simulink model "VehicleDynamics3D_old"  (R2018a)
settings: Solver=ode15s  StartTime=0.0  StopTime=Stoptime  FixedStep=.001  MaxStep=maxStep  RelTol=relTol  AbsTol=absTol  EnableMultiTasking=on
PreLoadFcn:
  | VehicleDynamicsInitialization.m
model workspace: external: MATLAB File C:\Users\Puspita\Desktop\VehicleDynamics\sm_suspension_templates_params_ori.m (data not in the file)
values from neighbouring files (symbols this model uses):
  contactDamping = 1200    [VehicleDynamicsInitialization.m]    (also in traj1_results.mat)
  contactStiffness = 1E+6    (= 1000000)    [VehicleDynamicsInitialization.m]    (also in traj1_results.mat)
  dwb =     [modelworkspace.mat]    (also in sm_suspension_templates_params_ref.m = struct)
  Floor =     [traj1_results.mat]
  followerCameraX = 7.5    [VehicleDynamicsInitialization.m]    (also in traj1_results.mat)
  followerCameraZ = 3    [VehicleDynamicsInitialization.m]    (also in traj1_results.mat)
  frontCameraX = -1.75    [VehicleDynamicsInitialization.m]    (also in traj1_results.mat)
  frontCameraZ = 0.35    [VehicleDynamicsInitialization.m]    (also in traj1_results.mat)
  isoCameraAimX = (1/2)*wheelbase    (= 0.75)    [VehicleDynamicsInitialization.m]    (also in traj1_results.mat)
  isoCameraX = -3.1    [VehicleDynamicsInitialization.m]    (also in traj1_results.mat)
  isoCameraY = 3.5    [VehicleDynamicsInitialization.m]    (also in traj1_results.mat)
  isoCameraZ = 1.5    [VehicleDynamicsInitialization.m]    (also in traj1_results.mat)
  kineticFrictionCoeff = 0.88    [VehicleDynamicsInitialization.m]    (also in traj1_results.mat)
  limit = 105    [Run_Rear_Ident.m]    (also in test_traj.m = 50; traj1_results.mat = 50)
  Load = 200*scale    (= 200)    [VehicleDynamicsInitialization.m]    (also in traj1_results.mat)
  m = 200    [test_2.mat]    (also in test_traj.mat; test_traj2.mat; traj1_results.mat; traj_8.mat)
  maxSteeringDisplacement = 12    [VehicleDynamicsInitialization.m]    (also in traj1_results.mat = 10)
  minSteeringDisplacement = -12    [VehicleDynamicsInitialization.m]    (also in traj1_results.mat = -10)
  SetPaceSampleTime = 0.1    [VehicleDynamicsInitialization.m]    (also in traj1_results.mat)
  staticFrictionCoeff = 0.90    (= 0.9)    [VehicleDynamicsInitialization.m]    (also in traj1_results.mat)
  steer_input_max = 10    [Run.m]    (also in Run_Front_Ident.m; Run_Rear_Ident.m = save_array(i,1); Run_Rear_Ident2.m)
  steering_step = 7.5/30    (= 0.25)    [Run.m]    (also in Run_Front_Ident.m; Run_Rear_Ident.m; Run_Rear_Ident2.m)
  steeringInput = 0    [VehicleDynamicsInitialization.m]    (also in traj1_results.mat)
  vehicleSpeed_kph = 0    [VehicleDynamicsInitialization.m]    (also in traj1_results.mat)
  velocityThreshold = 1.5    [VehicleDynamicsInitialization.m]    (also in traj1_results.mat)
  vx_input = vx_choice(i)    [Run.m]    (also in Run_Front_Ident.m; Run_Rear_Ident.m = save_array(i,2); Run_Rear_Ident2.m)
  wheel =     [modelworkspace.mat]    (also in sm_suspension_templates_params_ref.m = struct; traj1_results.mat)
  wheelbase = 1.5*scale    (= 1.5)    [VehicleDynamicsInitialization.m]    (also in traj1_results.mat)
undefined symbols (not defined in the file or in its folder): sigbuilder_block, X, Y, Z
libraries: sm_lib x235, nesl_utility x78, sm_suspension_templates_lib x34, Contact_Forces_Lib x16, simulink x12, fl_lib x1, aerolibanimutils x1
(part 7 of 10)

== system VehicleDynamics3D_old/WheelFR/FrontRightWeelContact ==
  Bus Selector : BusSelector  OutputSignals=Normal Force,Friction Force
  Demux : Demux  Outputs=2
  Math Function : Math  Operator=square  SaturateOnIntegerOverflow=on
  Rigid Transform : sm_lib/Frames and Transforms/Rigid Transform  TranslationMethod=StandardAxis  TranslationStandardOffset=-wheel.tire.outerradius*.01  TranslationLengthUnit=m  TranslationStandardAxis=+Z  TranslationCartesianOffset=[0 0 0]  TranslationROffset=0  TranslationROffsetUnits=m  TranslationZOffset=0  TranslationZOffsetUnits=m  TranslationThetaOffset=0  TranslationThetaOffsetUnits=deg  RotationMethod=None  RotationAngleUnits=deg  RotationStandardAxis=+Z  RotationAngle=0  RotationArbitraryAxis=[0 0 1]  FollAlignAxisA=+X  BaseAlignAxisA=-X  FollAlignAxisB=+Z  BaseAlignAxisB=+Z  RotationSequenceAxes=FollowerAxes  RotationSequence=XYX  RotationSequenceAngles=[0 0 0]  RotationSequenceAnglesUnits=deg  RotationMatrix=[1 0 0; 0 1 0; 0 0 1]
  Signal Conversion : SignalConversion  OverrideOpt=off
  Signal Conversion1 : SignalConversion  OverrideOpt=off
  Sphere to Plane Force : Subsystem  AncestorBlock=Contact_Forces_Lib/3D/Sphere to Plane Force  mask(Sphere to Plane Force){sphere_rad=wheel.tire.outerradius*.01, plane_lenx=Floor.l, plane_leny=Floor.w, plane_depth=Floor.h/2, force_law=Linear, k_contact=contactStiffness, b_contact=contactDamping, pen_full_damp_F=1e-4, pen_exponent=1, custom_param_1=1, custom_param_2=1, friction_law=Stick-Slip Continuous, mu_kinetic=kineticFrictionCoeff, mu_static=staticFrictionCoeff, v_thr=velocityThreshold, vis_on=off, vis_opc_en=0, vis_len_plaBz=0.005, vis_clr=[0.9 0.2 0.2], vis_opc=0.7}
      mask prompts: sphere_rad "Sphere Radius (m)"; plane_lenx "Plane Length x (m)"; plane_leny "Plane Length y (m)"; plane_depth "Plane Depth to Reference Frame (m)"; force_law "Force Law"; k_contact "Contact Stiffness (N/m)"; b_contact "Contact Damping (N/(m/s))"; pen_full_damp_F "Penetration for full damping (m)"; pen_exponent "Penetration exponent (>=1)"; custom_param_1 "Custom Parameter 1"; custom_param_2 "Custom Parameter 2"; friction_law "Friction Law"; mu_kinetic "Coefficient of Kinetic Friction"; mu_static "Coefficient of Static Friction"; v_thr "Velocity Threshold (m/s)"; vis_on "Visualize Contact Surfaces"; vis_opc_en "Visualize Opacity Enable"; vis_len_plaBz "Depth Plane Surface Element (Z-Axis) (m)"; vis_clr "Color of Surface Element (RGB)"; vis_opc "Opacity of Surface Element (0-1)"
      mask help:
      | This subsystem implements a contact force between a sphere and a plane.  The force is active above and below the plane.
      |
      | Frame connected to PlaB port:
      | 1. Located at midpoint of plane (x, y, and z).
      | 2. Z-axis is normal to the surfaces where force is active.
      |
      | Frame connected to the SphF port:
      | 1. Located at center of sphere.
      | 2. Orientation does not matter.
      |
      | Output signal is a bus with intermediate calculations and total force. Click Help for a diagram describing this force.
      mask init: same as VehicleDynamics3D_old/WheelFL/FrontLeftWeelContact/Sphere to Plane Force
      mask Help: web(which('Sphere_to_Plane_Contact.html'));
      mask TypeOptions force_law: Linear | Nonlinear | Custom
      mask Callback force_law:
      | %maskStr = get_param(gcb,'MaskValues');
      | maskObj = Simulink.Mask.get(gcb);
      | pfd_h = maskObj.getParameter('pen_full_damp_F');
      | pex_h = maskObj.getParameter('pen_exponent');
      | cc1_h = maskObj.getParameter('custom_param_1');
      | cc2_h = maskObj.getParameter('custom_param_2');
      | if strcmp(get_param(gcb,'force_law'),'Linear')
      |     pfd_h.Visible = 'off';
      |     pex_h.Visible = 'off';
      |     cc1_h.Visible = 'off';
      |     cc2_h.Visible = 'off';
      | %    set_param(gcb,'MaskVisibilities',{'on' 'on' 'on' 'on' 'on' 'off' 'off' 'off' 'off'});
      | %    set_param(gcb,'MaskVisibilities',{'on' 'on' 'on' 'on' 'on' 'off' 'off' 'off' 'off'});
      | elseif strcmp(get_param(gcb,'force_law'),'Nonlinear')
      |     pfd_h.Visible = 'on';
      |     pex_h.Visible = 'on';
      |     cc1_h.Visible = 'off';
      |     cc2_h.Visible = 'off';
      |     %set_param(gcb,'MaskVisibilities',{'on' 'on' 'on' 'on' 'on' 'on' 'on' 'off' 'off'});
      | elseif strcmp(get_param(gcb,'force_law'),'Custom')
      |     pfd_h.Visible = 'off';
      |     pex_h.Visible = 'off';
      |     cc1_h.Visible = 'on';
      |     cc2_h.Visible = 'on';
      |     %set_param(gcb,'MaskVisibilities',{'on' 'on' 'on' 'on' 'on' 'off' 'off' 'on' 'on'});
      | end
      | %clear maskObj
      | 
      | %maskObj = Simulink.Mask.get(gcb);
      | %if strcmp(get_param(gcb,'x'),'on')
      | %else
      | %    yh.Visible = 'off';
      | %end
      mask TypeOptions friction_law: None | Stick-Slip Continuous
      mask Callback friction_law:
      | maskObj = Simulink.Mask.get(gcb);
      | muk_h = maskObj.getParameter('mu_kinetic');
      | mus_h = maskObj.getParameter('mu_static');
      | vth_h = maskObj.getParameter('v_thr');
      | if strcmp(get_param(gcb,'friction_law'),'None')
      |     muk_h.Visible = 'off';
      |     mus_h.Visible = 'off';
      |     vth_h.Visible = 'off';
      | elseif strcmp(get_param(gcb,'friction_law'),'Stick-Slip Continuous')
      |     muk_h.Visible = 'on';
      |     mus_h.Visible = 'on';
      |     vth_h.Visible = 'on';
      | end
      | clear maskObj
      mask Callback vis_on:
      | maskObj = Simulink.Mask.get(gcb);
      | vis_clr_h = maskObj.getParameter('vis_clr');
      | vis_opc_h = maskObj.getParameter('vis_opc');
      | vis_len_plaBz_h = maskObj.getParameter('vis_len_plaBz');
      | if strcmp(get_param(gcb,'vis_on'),'off')
      |     vis_len_plaBz_h.Visible = 'off';
      |     vis_clr_h.Visible = 'off';
      |     vis_opc_h.Visible = 'off';
      | elseif strcmp(get_param(gcb,'vis_on'),'on')
      |     vis_len_plaBz_h.Visible = 'on';
      |     vis_clr_h.Visible = 'on';
      |     vis_opc_h.Visible = 'on';
      | end
      | clear maskObj vis_clr_h vis_opc_h
      | clear vis_len_plaBz_h
      mask DialogControl Dim_Cont Prompt: Dimensions
      mask DialogControl Con_Cont Prompt: Contact
      mask DialogControl Fri_Cont Prompt: Friction
      mask DialogControl Container9 Prompt: Visual
      mask Display: image('Sphere_to_Plane_Contact_IMAGE.jpg');
  Sqrt : Sqrt  SaturateOnIntegerOverflow=on
  Sum of Elements : Sum  Inputs=+
  Terminator : Terminator
  Terminator1 : Terminator
  Terminator2 : Terminator
  To Workspace2 : ToWorkspace  VariableName=F_Fr  SampleTime=-1
  Conn1 : PMIOPort  Side=Right
  Conn2 : PMIOPort  Port=2  Side=Left
  wires:
  Sphere to Plane Force/1(Out) -> Bus Selector/1  "FrontRight"
  Signal Conversion1/1 -> Terminator1/1  "FrontRightFriction"
  Bus Selector/1 -> Signal Conversion/1  "<Normal Force>"
  Sum of Elements/1 -> Sqrt/1
  Signal Conversion/1 -> Terminator/1  "FrontRightTireLoad"
  Math Function/1 -> Sum of Elements/1
  Bus Selector/2 -> Demux/1, Math Function/1  "<Friction Force>"
  Sqrt/1 -> Signal Conversion1/1
  Demux/1 -> To Workspace2/1
  Demux/2 -> Terminator2/1
  connections:
  Conn1/RConn1 -- Rigid Transform/RConn1
  Sphere to Plane Force/LConn1 -- Rigid Transform/LConn1
  Conn2/RConn1 -- Sphere to Plane Force/RConn1

== system VehicleDynamics3D_old/WheelRL/RearLeftWeelContact ==
  Bus Selector : BusSelector  OutputSignals=Normal Force,Friction Force
  Demux : Demux  Outputs=2
  Math Function : Math  Operator=square  SaturateOnIntegerOverflow=on
  Rigid Transform : sm_lib/Frames and Transforms/Rigid Transform  TranslationMethod=StandardAxis  TranslationStandardOffset=-wheel.tire.outerradius*.01  TranslationLengthUnit=m  TranslationStandardAxis=+Z  TranslationCartesianOffset=[0 0 0]  TranslationROffset=0  TranslationROffsetUnits=m  TranslationZOffset=0  TranslationZOffsetUnits=m  TranslationThetaOffset=0  TranslationThetaOffsetUnits=deg  RotationMethod=None  RotationAngleUnits=deg  RotationStandardAxis=+Z  RotationAngle=0  RotationArbitraryAxis=[0 0 1]  FollAlignAxisA=+X  BaseAlignAxisA=-X  FollAlignAxisB=+Z  BaseAlignAxisB=+Z  RotationSequenceAxes=FollowerAxes  RotationSequence=XYX  RotationSequenceAngles=[0 0 0]  RotationSequenceAnglesUnits=deg  RotationMatrix=[1 0 0; 0 1 0; 0 0 1]
  Signal Conversion : SignalConversion  OverrideOpt=off
  Signal Conversion1 : SignalConversion  OverrideOpt=off
  Sphere to Plane Force : Subsystem  AncestorBlock=Contact_Forces_Lib/3D/Sphere to Plane Force  mask(Sphere to Plane Force){sphere_rad=wheel.tire.outerradius*.01, plane_lenx=Floor.l, plane_leny=Floor.w, plane_depth=Floor.h/2, force_law=Linear, k_contact=contactStiffness, b_contact=contactDamping, pen_full_damp_F=1e-4, pen_exponent=1, custom_param_1=1, custom_param_2=1, friction_law=Stick-Slip Continuous, mu_kinetic=kineticFrictionCoeff, mu_static=staticFrictionCoeff, v_thr=velocityThreshold, vis_on=off, vis_opc_en=0, vis_len_plaBz=0.005, vis_clr=[0.9 0.2 0.2], vis_opc=0.7}
      mask prompts: sphere_rad "Sphere Radius (m)"; plane_lenx "Plane Length x (m)"; plane_leny "Plane Length y (m)"; plane_depth "Plane Depth to Reference Frame (m)"; force_law "Force Law"; k_contact "Contact Stiffness (N/m)"; b_contact "Contact Damping (N/(m/s))"; pen_full_damp_F "Penetration for full damping (m)"; pen_exponent "Penetration exponent (>=1)"; custom_param_1 "Custom Parameter 1"; custom_param_2 "Custom Parameter 2"; friction_law "Friction Law"; mu_kinetic "Coefficient of Kinetic Friction"; mu_static "Coefficient of Static Friction"; v_thr "Velocity Threshold (m/s)"; vis_on "Visualize Contact Surfaces"; vis_opc_en "Visualize Opacity Enable"; vis_len_plaBz "Depth Plane Surface Element (Z-Axis) (m)"; vis_clr "Color of Surface Element (RGB)"; vis_opc "Opacity of Surface Element (0-1)"
      mask help:
      | This subsystem implements a contact force between a sphere and a plane.  The force is active above and below the plane.
      |
      | Frame connected to PlaB port:
      | 1. Located at midpoint of plane (x, y, and z).
      | 2. Z-axis is normal to the surfaces where force is active.
      |
      | Frame connected to the SphF port:
      | 1. Located at center of sphere.
      | 2. Orientation does not matter.
      |
      | Output signal is a bus with intermediate calculations and total force. Click Help for a diagram describing this force.
      mask init: same as VehicleDynamics3D_old/WheelFL/FrontLeftWeelContact/Sphere to Plane Force
      mask Help: web(which('Sphere_to_Plane_Contact.html'));
      mask TypeOptions force_law: Linear | Nonlinear | Custom
      mask Callback force_law:
      | %maskStr = get_param(gcb,'MaskValues');
      | maskObj = Simulink.Mask.get(gcb);
      | pfd_h = maskObj.getParameter('pen_full_damp_F');
      | pex_h = maskObj.getParameter('pen_exponent');
      | cc1_h = maskObj.getParameter('custom_param_1');
      | cc2_h = maskObj.getParameter('custom_param_2');
      | if strcmp(get_param(gcb,'force_law'),'Linear')
      |     pfd_h.Visible = 'off';
      |     pex_h.Visible = 'off';
      |     cc1_h.Visible = 'off';
      |     cc2_h.Visible = 'off';
      | %    set_param(gcb,'MaskVisibilities',{'on' 'on' 'on' 'on' 'on' 'off' 'off' 'off' 'off'});
      | %    set_param(gcb,'MaskVisibilities',{'on' 'on' 'on' 'on' 'on' 'off' 'off' 'off' 'off'});
      | elseif strcmp(get_param(gcb,'force_law'),'Nonlinear')
      |     pfd_h.Visible = 'on';
      |     pex_h.Visible = 'on';
      |     cc1_h.Visible = 'off';
      |     cc2_h.Visible = 'off';
      |     %set_param(gcb,'MaskVisibilities',{'on' 'on' 'on' 'on' 'on' 'on' 'on' 'off' 'off'});
      | elseif strcmp(get_param(gcb,'force_law'),'Custom')
      |     pfd_h.Visible = 'off';
      |     pex_h.Visible = 'off';
      |     cc1_h.Visible = 'on';
      |     cc2_h.Visible = 'on';
      |     %set_param(gcb,'MaskVisibilities',{'on' 'on' 'on' 'on' 'on' 'off' 'off' 'on' 'on'});
      | end
      | %clear maskObj
      | 
      | %maskObj = Simulink.Mask.get(gcb);
      | %if strcmp(get_param(gcb,'x'),'on')
      | %else
      | %    yh.Visible = 'off';
      | %end
      mask TypeOptions friction_law: None | Stick-Slip Continuous
      mask Callback friction_law:
      | maskObj = Simulink.Mask.get(gcb);
      | muk_h = maskObj.getParameter('mu_kinetic');
      | mus_h = maskObj.getParameter('mu_static');
      | vth_h = maskObj.getParameter('v_thr');
      | if strcmp(get_param(gcb,'friction_law'),'None')
      |     muk_h.Visible = 'off';
      |     mus_h.Visible = 'off';
      |     vth_h.Visible = 'off';
      | elseif strcmp(get_param(gcb,'friction_law'),'Stick-Slip Continuous')
      |     muk_h.Visible = 'on';
      |     mus_h.Visible = 'on';
      |     vth_h.Visible = 'on';
      | end
      | clear maskObj
      mask Callback vis_on:
      | maskObj = Simulink.Mask.get(gcb);
      | vis_clr_h = maskObj.getParameter('vis_clr');
      | vis_opc_h = maskObj.getParameter('vis_opc');
      | vis_len_plaBz_h = maskObj.getParameter('vis_len_plaBz');
      | if strcmp(get_param(gcb,'vis_on'),'off')
      |     vis_len_plaBz_h.Visible = 'off';
      |     vis_clr_h.Visible = 'off';
      |     vis_opc_h.Visible = 'off';
      | elseif strcmp(get_param(gcb,'vis_on'),'on')
      |     vis_len_plaBz_h.Visible = 'on';
      |     vis_clr_h.Visible = 'on';
      |     vis_opc_h.Visible = 'on';
      | end
      | clear maskObj vis_clr_h vis_opc_h
      | clear vis_len_plaBz_h
      mask DialogControl Dim_Cont Prompt: Dimensions
      mask DialogControl Con_Cont Prompt: Contact
      mask DialogControl Fri_Cont Prompt: Friction
      mask DialogControl Container9 Prompt: Visual
      mask Display: image('Sphere_to_Plane_Contact_IMAGE.jpg');
  Sqrt : Sqrt  SaturateOnIntegerOverflow=on
  Sum of Elements : Sum  Inputs=+
  Terminator : Terminator
  Terminator1 : Terminator
  Terminator2 : Terminator
  To Workspace2 : ToWorkspace  VariableName=F_Rl  SampleTime=-1
  Conn1 : PMIOPort  Side=Right
  Conn2 : PMIOPort  Port=2  Side=Left
  wires:
  Sphere to Plane Force/1(Out) -> Bus Selector/1
  Signal Conversion1/1 -> Terminator2/1  "RearLeftFriction"
  Sum of Elements/1 -> Sqrt/1
  Bus Selector/1 -> Signal Conversion/1  "<Normal Force>"
  Signal Conversion/1 -> Terminator/1  "RearLeftTireLoad"
  Math Function/1 -> Sum of Elements/1
  Sqrt/1 -> Signal Conversion1/1
  Bus Selector/2 -> Demux/1, Math Function/1  "<Friction Force>"
  Demux/1 -> To Workspace2/1
  Demux/2 -> Terminator1/1
  connections:
  Conn1/RConn1 -- Rigid Transform/RConn1
  Sphere to Plane Force/LConn1 -- Rigid Transform/LConn1
  Sphere to Plane Force/RConn1 -- Conn2/RConn1

== system VehicleDynamics3D_old/WheelRR/RearRightWeelContact ==
  Bus Selector : BusSelector  OutputSignals=Normal Force,Friction Force
  Demux : Demux  Outputs=2
  Math Function : Math  Operator=square  SaturateOnIntegerOverflow=on
  Rigid Transform : sm_lib/Frames and Transforms/Rigid Transform  TranslationMethod=StandardAxis  TranslationStandardOffset=-wheel.tire.outerradius*.01  TranslationLengthUnit=m  TranslationStandardAxis=+Z  TranslationCartesianOffset=[0 0 0]  TranslationROffset=0  TranslationROffsetUnits=m  TranslationZOffset=0  TranslationZOffsetUnits=m  TranslationThetaOffset=0  TranslationThetaOffsetUnits=deg  RotationMethod=None  RotationAngleUnits=deg  RotationStandardAxis=+Z  RotationAngle=0  RotationArbitraryAxis=[0 0 1]  FollAlignAxisA=+X  BaseAlignAxisA=-X  FollAlignAxisB=+Z  BaseAlignAxisB=+Z  RotationSequenceAxes=FollowerAxes  RotationSequence=XYX  RotationSequenceAngles=[0 0 0]  RotationSequenceAnglesUnits=deg  RotationMatrix=[1 0 0; 0 1 0; 0 0 1]
  Signal Conversion : SignalConversion  OverrideOpt=off
  Signal Conversion1 : SignalConversion  OverrideOpt=off
  Sphere to Plane Force : Subsystem  AncestorBlock=Contact_Forces_Lib/3D/Sphere to Plane Force  mask(Sphere to Plane Force){sphere_rad=wheel.tire.outerradius*.01, plane_lenx=Floor.l, plane_leny=Floor.w, plane_depth=Floor.h/2, force_law=Linear, k_contact=contactStiffness, b_contact=contactDamping, pen_full_damp_F=1e-4, pen_exponent=1, custom_param_1=1, custom_param_2=1, friction_law=Stick-Slip Continuous, mu_kinetic=kineticFrictionCoeff, mu_static=staticFrictionCoeff, v_thr=velocityThreshold, vis_on=off, vis_opc_en=0, vis_len_plaBz=0.005, vis_clr=[0.9 0.2 0.2], vis_opc=0.7}
      mask prompts: sphere_rad "Sphere Radius (m)"; plane_lenx "Plane Length x (m)"; plane_leny "Plane Length y (m)"; plane_depth "Plane Depth to Reference Frame (m)"; force_law "Force Law"; k_contact "Contact Stiffness (N/m)"; b_contact "Contact Damping (N/(m/s))"; pen_full_damp_F "Penetration for full damping (m)"; pen_exponent "Penetration exponent (>=1)"; custom_param_1 "Custom Parameter 1"; custom_param_2 "Custom Parameter 2"; friction_law "Friction Law"; mu_kinetic "Coefficient of Kinetic Friction"; mu_static "Coefficient of Static Friction"; v_thr "Velocity Threshold (m/s)"; vis_on "Visualize Contact Surfaces"; vis_opc_en "Visualize Opacity Enable"; vis_len_plaBz "Depth Plane Surface Element (Z-Axis) (m)"; vis_clr "Color of Surface Element (RGB)"; vis_opc "Opacity of Surface Element (0-1)"
      mask help:
      | This subsystem implements a contact force between a sphere and a plane.  The force is active above and below the plane.
      |
      | Frame connected to PlaB port:
      | 1. Located at midpoint of plane (x, y, and z).
      | 2. Z-axis is normal to the surfaces where force is active.
      |
      | Frame connected to the SphF port:
      | 1. Located at center of sphere.
      | 2. Orientation does not matter.
      |
      | Output signal is a bus with intermediate calculations and total force. Click Help for a diagram describing this force.
      mask init: same as VehicleDynamics3D_old/WheelFL/FrontLeftWeelContact/Sphere to Plane Force
      mask Help: web(which('Sphere_to_Plane_Contact.html'));
      mask TypeOptions force_law: Linear | Nonlinear | Custom
      mask Callback force_law:
      | %maskStr = get_param(gcb,'MaskValues');
      | maskObj = Simulink.Mask.get(gcb);
      | pfd_h = maskObj.getParameter('pen_full_damp_F');
      | pex_h = maskObj.getParameter('pen_exponent');
      | cc1_h = maskObj.getParameter('custom_param_1');
      | cc2_h = maskObj.getParameter('custom_param_2');
      | if strcmp(get_param(gcb,'force_law'),'Linear')
      |     pfd_h.Visible = 'off';
      |     pex_h.Visible = 'off';
      |     cc1_h.Visible = 'off';
      |     cc2_h.Visible = 'off';
      | %    set_param(gcb,'MaskVisibilities',{'on' 'on' 'on' 'on' 'on' 'off' 'off' 'off' 'off'});
      | %    set_param(gcb,'MaskVisibilities',{'on' 'on' 'on' 'on' 'on' 'off' 'off' 'off' 'off'});
      | elseif strcmp(get_param(gcb,'force_law'),'Nonlinear')
      |     pfd_h.Visible = 'on';
      |     pex_h.Visible = 'on';
      |     cc1_h.Visible = 'off';
      |     cc2_h.Visible = 'off';
      |     %set_param(gcb,'MaskVisibilities',{'on' 'on' 'on' 'on' 'on' 'on' 'on' 'off' 'off'});
      | elseif strcmp(get_param(gcb,'force_law'),'Custom')
      |     pfd_h.Visible = 'off';
      |     pex_h.Visible = 'off';
      |     cc1_h.Visible = 'on';
      |     cc2_h.Visible = 'on';
      |     %set_param(gcb,'MaskVisibilities',{'on' 'on' 'on' 'on' 'on' 'off' 'off' 'on' 'on'});
      | end
      | %clear maskObj
      | 
      | %maskObj = Simulink.Mask.get(gcb);
      | %if strcmp(get_param(gcb,'x'),'on')
      | %else
      | %    yh.Visible = 'off';
      | %end
      mask TypeOptions friction_law: None | Stick-Slip Continuous
      mask Callback friction_law:
      | maskObj = Simulink.Mask.get(gcb);
      | muk_h = maskObj.getParameter('mu_kinetic');
      | mus_h = maskObj.getParameter('mu_static');
      | vth_h = maskObj.getParameter('v_thr');
      | if strcmp(get_param(gcb,'friction_law'),'None')
      |     muk_h.Visible = 'off';
      |     mus_h.Visible = 'off';
      |     vth_h.Visible = 'off';
      | elseif strcmp(get_param(gcb,'friction_law'),'Stick-Slip Continuous')
      |     muk_h.Visible = 'on';
      |     mus_h.Visible = 'on';
      |     vth_h.Visible = 'on';
      | end
      | clear maskObj
      mask Callback vis_on:
      | maskObj = Simulink.Mask.get(gcb);
      | vis_clr_h = maskObj.getParameter('vis_clr');
      | vis_opc_h = maskObj.getParameter('vis_opc');
      | vis_len_plaBz_h = maskObj.getParameter('vis_len_plaBz');
      | if strcmp(get_param(gcb,'vis_on'),'off')
      |     vis_len_plaBz_h.Visible = 'off';
      |     vis_clr_h.Visible = 'off';
      |     vis_opc_h.Visible = 'off';
      | elseif strcmp(get_param(gcb,'vis_on'),'on')
      |     vis_len_plaBz_h.Visible = 'on';
      |     vis_clr_h.Visible = 'on';
      |     vis_opc_h.Visible = 'on';
      | end
      | clear maskObj vis_clr_h vis_opc_h
      | clear vis_len_plaBz_h
      mask DialogControl Dim_Cont Prompt: Dimensions
      mask DialogControl Con_Cont Prompt: Contact
      mask DialogControl Fri_Cont Prompt: Friction
      mask DialogControl Container9 Prompt: Visual
      mask Display: image('Sphere_to_Plane_Contact_IMAGE.jpg');
  Sqrt : Sqrt  SaturateOnIntegerOverflow=on
  Sum of Elements : Sum  Inputs=+
  Terminator1 : Terminator
  Terminator2 : Terminator
  Terminator3 : Terminator
  To Workspace2 : ToWorkspace  VariableName=F_Rr  SampleTime=-1
  Conn1 : PMIOPort  Side=Right
  Conn2 : PMIOPort  Port=2  Side=Left
  wires:
  Sphere to Plane Force/1(Out) -> Bus Selector/1  "RearRight"
  Bus Selector/1 -> Signal Conversion1/1  "<Normal Force>"
  Bus Selector/2 -> Demux/1, Signal Conversion/1  "<Friction Force>"
  Math Function/1 -> Sum of Elements/1
  Sum of Elements/1 -> Sqrt/1
  Sqrt/1 -> Terminator2/1  "RearRightFriction"
  Signal Conversion/1 -> Math Function/1
  Signal Conversion1/1 -> Terminator1/1  "RearRightTireLoad"
  Demux/1 -> To Workspace2/1
  Demux/2 -> Terminator3/1
  connections:
  Sphere to Plane Force/LConn1 -- Rigid Transform/LConn1
  Conn1/RConn1 -- Rigid Transform/RConn1
  Conn2/RConn1 -- Sphere to Plane Force/RConn1

== system VehicleDynamics3D_old/FrontSuspension/6DOF Motion/WraptTo180 ==
  Yaw : Inport
  Bias : Bias  Bias=-180
  Bias1 : Bias  Bias=180
  Constant : Constant  Value=360
  Interval Test : simulink/Logic and Bit Operations/Interval Test  IntervalClosedRight=on  uplimit=180  IntervalClosedLeft=off  lowlimit=-180  OutDataTypeStr=boolean
  Math Function : Math  Operator=mod  SaturateOnIntegerOverflow=on
  Switch : Switch  Criteria=u2 ~= 0
  NormalizedYaw : Outport
  wires:
  Bias1/1 -> Math Function/1
  Switch/1 -> NormalizedYaw/1  "VehicleYawNormalized_Deg"
  Constant/1 -> Math Function/2
  Interval Test/1 -> Switch/2
  Math Function/1 -> Bias/1
  Bias/1 -> Switch/3
  Yaw/1 -> Switch/1, Interval Test/1, Bias1/1

== system VehicleDynamics3D_old/FrontSuspension/Chassis Assembly/Front Frame ==
  DL XForm : sm_lib/Frames and Transforms/Rigid Transform  TranslationMethod=Cartesian  TranslationStandardOffset=0  TranslationLengthUnit=cm  TranslationStandardAxis=+Z  TranslationCartesianOffset=[swc 0]  TranslationROffset=0  TranslationROffsetUnits=m  TranslationZOffset=0  TranslationZOffsetUnits=m  TranslationThetaOffset=0  TranslationThetaOffsetUnits=deg  RotationMethod=None  RotationAngleUnits=deg  RotationStandardAxis=+Z  RotationAngle=0  RotationArbitraryAxis=[0 0 1]  FollAlignAxisA=+X  BaseAlignAxisA=-X  FollAlignAxisB=+Y  BaseAlignAxisB=-Y  RotationSequenceAxes=FollowerAxes  RotationSequence=XYX  RotationSequenceAngles=[0 0 0]  RotationSequenceAnglesUnits=deg  RotationMatrix=[1 0 0; 0 1 0; 0 0 1]
  DR XForm : sm_lib/Frames and Transforms/Rigid Transform  TranslationMethod=Cartesian  TranslationStandardOffset=0  TranslationLengthUnit=cm  TranslationStandardAxis=+Z  TranslationCartesianOffset=[sec 0]  TranslationROffset=0  TranslationROffsetUnits=m  TranslationZOffset=0  TranslationZOffsetUnits=m  TranslationThetaOffset=0  TranslationThetaOffsetUnits=deg  RotationMethod=None  RotationAngleUnits=deg  RotationStandardAxis=+Z  RotationAngle=0  RotationArbitraryAxis=[0 0 1]  FollAlignAxisA=+X  BaseAlignAxisA=+Y  FollAlignAxisB=+Y  BaseAlignAxisB=+Z  RotationSequenceAxes=FollowerAxes  RotationSequence=XYX  RotationSequenceAngles=[0 0 0]  RotationSequenceAnglesUnits=deg  RotationMatrix=[1 0 0; 0 1 0; 0 0 1]
  Frame : sm_lib/Body Elements/Solid  InertiaType=CalculateFromGeometry  Mass=1  MassUnits=kg  CenterOfMass=[0 0 0]  CenterOfMassUnits=m  MomentsOfInertia=[1 1 1]  MomentsOfInertiaUnits=kg*m^2  ProductsOfInertia=[0 0 0]  ProductsOfInertiaUnits=kg*m^2  DensityBased=on  Density=rho  DensityUnits=kg/(m^3)  DoExposeReferenceFrame=on  SerializedFrames=<Frames/>  GraphicType=FromGeometry  MarkerShape=Sphere  MarkerSize=10  MarkerSizeUnits=m  GraphicVisPropType=SimpleVisualProperties  GraphicDiffuseColor=clr  GraphicSpecularColor=[0.5 0.5 0.5 1.0]  GraphicAmbientColor=[0.15 0.15 0.15 1.0]  GraphicEmissiveColor=[0.0 0.0 0.0 1.0]  GraphicShininess=75  GraphicOpacity=1.0  GeometryShape=GeneralExtrusion  RectangleSize=[1 1]  RectangleSizeUnits=m  BrickDimensions=[1 1 1]  BrickDimensionUnits=m  CylinderRadius=1  CylinderRadiusUnits=m  CylinderLength=1  CylinderLengthUnits=m  SphereRadius=1  SphereRadiusUnits=m  EllipsoidRadii=[1 1 1]  EllipsoidRadiiUnits=m  ExtrusionCrossSection=frame_xsec  ExtrusionCrossSectionUnits=cm  ExtrusionLength=T  ExtrusionLengthUnits=cm  PolygonNumSides=3  PolygonOuterRadius=1  PolygonOuterRadiusUnits=m  ExtGeomFileType=STL  ExtGeomFileUnits=m  RevolutionCrossSection=[1 1; 1 -1; 2 -1; 2 1]  RevolutionCrossSectionUnits=m  RevolutionExtent=Full  RevolutionAngle=180  RevolutionAngleUnits=deg
  UL XForm : sm_lib/Frames and Transforms/Rigid Transform  TranslationMethod=Cartesian  TranslationStandardOffset=0  TranslationLengthUnit=cm  TranslationStandardAxis=+Z  TranslationCartesianOffset=[nwc 0]  TranslationROffset=0  TranslationROffsetUnits=m  TranslationZOffset=0  TranslationZOffsetUnits=m  TranslationThetaOffset=0  TranslationThetaOffsetUnits=deg  RotationMethod=None  RotationAngleUnits=deg  RotationStandardAxis=+Z  RotationAngle=0  RotationArbitraryAxis=[0 0 1]  FollAlignAxisA=+X  BaseAlignAxisA=-X  FollAlignAxisB=+Y  BaseAlignAxisB=-Y  RotationSequenceAxes=FollowerAxes  RotationSequence=XYX  RotationSequenceAngles=[0 0 0]  RotationSequenceAnglesUnits=deg  RotationMatrix=[1 0 0; 0 1 0; 0 0 1]
  UR XForm : sm_lib/Frames and Transforms/Rigid Transform  TranslationMethod=Cartesian  TranslationStandardOffset=0  TranslationLengthUnit=cm  TranslationStandardAxis=+Z  TranslationCartesianOffset=[nec 0]  TranslationROffset=0  TranslationROffsetUnits=m  TranslationZOffset=0  TranslationZOffsetUnits=m  TranslationThetaOffset=0  TranslationThetaOffsetUnits=deg  RotationMethod=None  RotationAngleUnits=deg  RotationStandardAxis=+Z  RotationAngle=0  RotationArbitraryAxis=[0 0 1]  FollAlignAxisA=+X  BaseAlignAxisA=+Y  FollAlignAxisB=+Y  BaseAlignAxisB=+Z  RotationSequenceAxes=FollowerAxes  RotationSequence=XYX  RotationSequenceAngles=[0 0 0]  RotationSequenceAnglesUnits=deg  RotationMatrix=[1 0 0; 0 1 0; 0 0 1]
  UL : PMIOPort  Side=Left
  DL : PMIOPort  Port=2  Side=Left
  DR : PMIOPort  Port=3  Side=Left
  UR : PMIOPort  Port=4  Side=Left
  connections:
  Frame/RConn1 -- UL XForm/LConn1 -- DL XForm/LConn1 -- DR XForm/LConn1 -- UR XForm/LConn1
  UR XForm/RConn1 -- UR/RConn1
  DL XForm/RConn1 -- DL/RConn1
  UL XForm/RConn1 -- UL/RConn1
  DR XForm/RConn1 -- DR/RConn1

== system VehicleDynamics3D_old/FrontSuspension/Chassis Assembly/Load ==
  Chassis Load : sm_lib/Body Elements/Solid  InertiaType=PointMass  Mass=Load  MassUnits=kg  CenterOfMass=[0 0 0]  CenterOfMassUnits=m  MomentsOfInertia=[1 1 1]  MomentsOfInertiaUnits=kg*m^2  ProductsOfInertia=[0 0 0]  ProductsOfInertiaUnits=kg*m^2  DensityBased=off  Density=1000  DensityUnits=kg/(m^3)  DoExposeReferenceFrame=on  SerializedFrames=<Frames/>  GraphicType=FromGeometry  MarkerShape=Sphere  MarkerSize=10  MarkerSizeUnits=m  GraphicVisPropType=SimpleVisualProperties  GraphicDiffuseColor=[0.6 0.0 0.0]  GraphicSpecularColor=[0.5 0.5 0.5 1.0]  GraphicAmbientColor=[0.15 0.15 0.15 1.0]  GraphicEmissiveColor=[0.0 0.0 0.0 1.0]  GraphicShininess=75  GraphicOpacity=1.0  GeometryShape=Brick  RectangleSize=[1 1]  RectangleSizeUnits=m  BrickDimensions=[5 5 5]  BrickDimensionUnits=cm  CylinderRadius=1  CylinderRadiusUnits=m  CylinderLength=1  CylinderLengthUnits=m  SphereRadius=1  SphereRadiusUnits=m  EllipsoidRadii=[1 1 1]  EllipsoidRadiiUnits=m  ExtrusionCrossSection=[1 1; -1 1; -1 -1; 1 -1]  ExtrusionCrossSectionUnits=m  ExtrusionLength=1  ExtrusionLengthUnits=m  PolygonNumSides=3  PolygonOuterRadius=1  PolygonOuterRadiusUnits=m  ExtGeomFileType=STL  ExtGeomFileUnits=m  RevolutionCrossSection=[1 1; 1 -1; 2 -1; 2 1]  RevolutionCrossSectionUnits=m  RevolutionExtent=Full  RevolutionAngle=180  RevolutionAngleUnits=deg
  Chassis Load XForm : sm_lib/Frames and Transforms/Rigid Transform  TranslationMethod=StandardAxis  TranslationStandardOffset=15  TranslationLengthUnit=cm  TranslationStandardAxis=+X  TranslationCartesianOffset=[0 0 0]  TranslationROffset=0  TranslationROffsetUnits=m  TranslationZOffset=0  TranslationZOffsetUnits=m  TranslationThetaOffset=0  TranslationThetaOffsetUnits=deg  RotationMethod=None  RotationAngleUnits=deg  RotationStandardAxis=+Z  RotationAngle=0  RotationArbitraryAxis=[0 0 1]  FollAlignAxisA=+X  BaseAlignAxisA=+Y  FollAlignAxisB=+Y  BaseAlignAxisB=+Z  RotationSequenceAxes=FollowerAxes  RotationSequence=XYX  RotationSequenceAngles=[0 0 0]  RotationSequenceAnglesUnits=deg  RotationMatrix=[1 0 0; 0 1 0; 0 0 1]
  L : PMIOPort  Side=Right
  connections:
  Chassis Load XForm/LConn1 -- L/RConn1
  Chassis Load/RConn1 -- Chassis Load XForm/RConn1

== system VehicleDynamics3D_old/FrontSuspension/Chassis Assembly/Steering System ==
  L Rack Bracket : sm_suspension_templates_lib/Rectangular Hole Bracket  L=dwb.chassis.steering.bracket.length  W=dwb.chassis.steering.bracket.width  T=dwb.chassis.steering.bracket.thickness  Lh=dwb.chassis.steering.bracket.holelength  Wh=dwb.chassis.steering.bracket.holewidth  Rr=dwb.chassis.steering.bracket.chamferradius  rho=dwb.chassis.steering.bracket.density  clr=dwb.chassis.steering.bracket.color
  L Rack Bracket XForm : sm_lib/Frames and Transforms/Rigid Transform  TranslationMethod=Cartesian  TranslationStandardOffset=0  TranslationLengthUnit=cm  TranslationStandardAxis=+X  TranslationCartesianOffset=[-1 -35 -18]  TranslationROffset=0  TranslationROffsetUnits=m  TranslationZOffset=0  TranslationZOffsetUnits=m  TranslationThetaOffset=0  TranslationThetaOffsetUnits=deg  RotationMethod=AlignedAxes  RotationAngleUnits=deg  RotationStandardAxis=+Z  RotationAngle=0  RotationArbitraryAxis=[0 0 1]  FollAlignAxisA=+Z  BaseAlignAxisA=-X  FollAlignAxisB=+X  BaseAlignAxisB=-Z  RotationSequenceAxes=FollowerAxes  RotationSequence=XYX  RotationSequenceAngles=[0 0 0]  RotationSequenceAnglesUnits=deg  RotationMatrix=[1 0 0; 0 1 0; 0 0 1]
  L Tie Rod : sm_suspension_templates_lib/Tie Rod  L=dwb.chassis.steering.tierod.rod.length  R=dwb.chassis.steering.tierod.rod.radius  Rr=dwb.chassis.steering.tierod.rod.chamferradius  Lb=dwb.chassis.steering.tierod.bracket.length  Wb=dwb.chassis.steering.tierod.bracket.width  Tb=dwb.chassis.steering.tierod.bracket.thickness  Sb=dwb.chassis.steering.tierod.bracket.flangespacing  Rs=dwb.chassis.steering.tierod.bracket.socketradius  Rb=dwb.chassis.steering.tierod.bracket.ballradius  Rh=dwb.chassis.steering.tierod.bracket.holeradius  rho=dwb.chassis.steering.tierod.density  tclr=dwb.chassis.steering.tierod.rod.color  bclr=dwb.chassis.steering.tierod.ballcolor
  LBR Joint : sm_lib/Joints/Prismatic Joint  SenseConstraintForce=off  SenseConstraintForceX=off  SenseConstraintForceY=off  SenseConstraintForceZ=off  SenseConstraintTorque=off  SenseConstraintTorqueX=off  SenseConstraintTorqueY=off  SenseConstraintTorqueZ=off  SenseTotalForce=off  SenseTotalForceX=off  SenseTotalForceY=off  SenseTotalForceZ=off  SenseTotalTorque=off  SenseTotalTorqueX=off  SenseTotalTorqueY=off  SenseTotalTorqueZ=off  CompositeWrenchDir=FollowerOnBase  CompositeWrenchFrame=BaseFrame  EquilibriumPosition=0  EquilibriumPositionUnits=m  SpringStiffness=steeringJointStiffness  SpringStiffnessUnits=N/m  DampingCoefficient=steeringJointDamping  DampingCoefficientUnits=N/(m/s)  TorqueActuationMode=ComputedTorque  MotionActuationMode=InputMotion  SensePosition=off  SenseVelocity=off  SenseAcceleration=off  SenseTorqueForce=off  PositionTargetSpecify=on  PositionTargetPriority=High  PositionTargetValue=0  PositionTargetValueUnits=cm  VelocityTargetSpecify=off  VelocityTargetPriority=High  VelocityTargetValue=0  VelocityTargetValueUnits=m/s
  LRTie Joint : sm_lib/Joints/Revolute Joint  SenseConstraintForce=off  SenseConstraintForceX=off  SenseConstraintForceY=off  SenseConstraintForceZ=off  SenseConstraintTorque=off  SenseConstraintTorqueX=off  SenseConstraintTorqueY=off  SenseConstraintTorqueZ=off  SenseTotalForce=off  SenseTotalForceX=off  SenseTotalForceY=off  SenseTotalForceZ=off  SenseTotalTorque=off  SenseTotalTorqueX=off  SenseTotalTorqueY=off  SenseTotalTorqueZ=off  CompositeWrenchDir=FollowerOnBase  CompositeWrenchFrame=BaseFrame  EquilibriumPosition=0  EquilibriumPositionUnits=deg  SpringStiffness=0  SpringStiffnessUnits=N*m/deg  DampingCoefficient=0  DampingCoefficientUnits=N*m/(deg/s)  TorqueActuationMode=NoTorque  MotionActuationMode=ComputedMotion  SensePosition=off  SenseVelocity=off  SenseAcceleration=off  SenseTorqueForce=off  PositionTargetSpecify=on  PositionTargetPriority=Low  PositionTargetValue=160  PositionTargetValueUnits=deg  VelocityTargetSpecify=off  VelocityTargetPriority=High  VelocityTargetValue=0  VelocityTargetValueUnits=deg/s
  R Rack Bracket : sm_suspension_templates_lib/Rectangular Hole Bracket  L=dwb.chassis.steering.bracket.length  W=dwb.chassis.steering.bracket.width  T=dwb.chassis.steering.bracket.thickness  Lh=dwb.chassis.steering.bracket.holelength  Wh=dwb.chassis.steering.bracket.holewidth  Rr=dwb.chassis.steering.bracket.chamferradius  rho=dwb.chassis.steering.bracket.density  clr=dwb.chassis.steering.bracket.color
  R Rack Bracket XForm : sm_lib/Frames and Transforms/Rigid Transform  TranslationMethod=Cartesian  TranslationStandardOffset=0  TranslationLengthUnit=cm  TranslationStandardAxis=-X  TranslationCartesianOffset=[-1 35 -18]  TranslationROffset=0  TranslationROffsetUnits=m  TranslationZOffset=0  TranslationZOffsetUnits=m  TranslationThetaOffset=0  TranslationThetaOffsetUnits=deg  RotationMethod=AlignedAxes  RotationAngleUnits=deg  RotationStandardAxis=+Z  RotationAngle=0  RotationArbitraryAxis=[0 0 1]  FollAlignAxisA=+Z  BaseAlignAxisA=-X  FollAlignAxisB=+X  BaseAlignAxisB=-Z  RotationSequenceAxes=FollowerAxes  RotationSequence=XYX  RotationSequenceAngles=[0 0 0]  RotationSequenceAnglesUnits=deg  RotationMatrix=[1 0 0; 0 1 0; 0 0 1]
  R Tie Rod : sm_suspension_templates_lib/Tie Rod  L=dwb.chassis.steering.tierod.rod.length  R=dwb.chassis.steering.tierod.rod.radius  Rr=dwb.chassis.steering.tierod.rod.chamferradius  Lb=dwb.chassis.steering.tierod.bracket.length  Wb=dwb.chassis.steering.tierod.bracket.width  Tb=dwb.chassis.steering.tierod.bracket.thickness  Sb=dwb.chassis.steering.tierod.bracket.flangespacing  Rs=dwb.chassis.steering.tierod.bracket.socketradius  Rb=dwb.chassis.steering.tierod.bracket.ballradius  Rh=dwb.chassis.steering.tierod.bracket.holeradius  rho=dwb.chassis.steering.tierod.density  tclr=dwb.chassis.steering.tierod.rod.color  bclr=dwb.chassis.steering.tierod.ballcolor
  RRTie Joint : sm_lib/Joints/Revolute Joint  SenseConstraintForce=off  SenseConstraintForceX=off  SenseConstraintForceY=off  SenseConstraintForceZ=off  SenseConstraintTorque=off  SenseConstraintTorqueX=off  SenseConstraintTorqueY=off  SenseConstraintTorqueZ=off  SenseTotalForce=off  SenseTotalForceX=off  SenseTotalForceY=off  SenseTotalForceZ=off  SenseTotalTorque=off  SenseTotalTorqueX=off  SenseTotalTorqueY=off  SenseTotalTorqueZ=off  CompositeWrenchDir=FollowerOnBase  CompositeWrenchFrame=BaseFrame  EquilibriumPosition=0  EquilibriumPositionUnits=deg  SpringStiffness=0  SpringStiffnessUnits=N*m/deg  DampingCoefficient=0  DampingCoefficientUnits=N*m/(deg/s)  TorqueActuationMode=NoTorque  MotionActuationMode=ComputedMotion  SensePosition=off  SenseVelocity=off  SenseAcceleration=off  SenseTorqueForce=off  PositionTargetSpecify=on  PositionTargetPriority=Low  PositionTargetValue=160  PositionTargetValueUnits=deg  VelocityTargetSpecify=off  VelocityTargetPriority=High  VelocityTargetValue=0  VelocityTargetValueUnits=deg/s
  Steer Rack : Subsystem  mask(Steering Rack){L=dwb.chassis.steering.rack.rod.length, W=dwb.chassis.steering.rack.rod.width, H=dwb.chassis.steering.rack.rod.height, Db=dwb.chassis.steering.rack.rod.bracketdistance, Rr=dwb.chassis.steering.rack.rod.chamferradius, Lb=dwb.chassis.steering.rack.bracket.length, Wb=dwb.chassis.steering.rack.bracket.width, Tb=dwb.chassis.steering.rack.bracket.thickness, Rh=dwb.chassis.steering.rack.bracket.holeradius, rho=dwb.chassis.steering.rack.density, clr=dwb.chassis.steering.rack.color}
      mask prompts: L "Length (cm):"; W "Width (cm):"; H "Height (cm):"; Db "Distance between holding brackets (cm):"; Rr "Chamfer/fillet radius (cm):"; Lb "Length (cm):"; Wb "Width (cm):"; Tb "Thickness (cm):"; Rh "Hole radius (cm):"; rho "Density (kg/m^3):"; clr "Color ([r g b]):"
      mask help: This block models a steering rack with brackets at the end that connect to tie rods. The ports LT and RT correspond to the left and right tie rod frames. The ports LB and RB refer to the left and right holding bracket frames.
      mask init:
      | rack_xsec = [W/2 -H/2; W/2 H/2; -W/2 H/2; -W/2 -H/2];
      | rack_xsec = simmechanics.demohelpers.round_corners(rack_xsec,1:4,Rr,5);
      mask DialogControl ParameterTabVar0 Prompt: Rod
      mask DialogControl ParameterTabVar01 Prompt: Brackets
      mask DialogControl ParameterTabVar012 Prompt: Material Properties
      mask Display:
      | image(imread(fullfile(matlabroot,...
      |     'toolbox','physmod','sm','smdemos',...
      |     'suspension_templates','images','sm_isuspension_steerrack.png')));
      | 
      | port_label('LConn',1,'LB');
      | port_label('LConn',2,'LT');
      | port_label('RConn',1,'RB');
      | port_label('RConn',2,'RT');
  BC : PMIOPort  Side=Left
  LT : PMIOPort  Port=2  Side=Right
  RT : PMIOPort  Port=3  Side=Right
  S : PMIOPort  Port=4  Side=Left
  connections:
  LBR Joint/RConn1 -- Steer Rack/LConn1
  R Rack Bracket/LConn1 -- R Rack Bracket XForm/RConn1
  Steer Rack/RConn2 -- RRTie Joint/LConn1
  R Tie Rod/RConn1 -- RT/RConn1
  LRTie Joint/LConn1 -- Steer Rack/LConn2
  LBR Joint/LConn1 -- L Rack Bracket/RConn1
  L Tie Rod/LConn1 -- LRTie Joint/RConn1
  LT/RConn1 -- L Tie Rod/RConn1
  RRTie Joint/RConn1 -- R Tie Rod/LConn1
  L Rack Bracket/LConn1 -- L Rack Bracket XForm/RConn1
  L Rack Bracket XForm/LConn1 -- BC/RConn1 -- R Rack Bracket XForm/LConn1
  S/RConn1 -- LBR Joint/LConn2

== system VehicleDynamics3D_old/Inputs/SpeedProcessing/mps2mph ==
  V[kph] : Inport
  Signal Specification : SignalSpecification  Unit=m/s
  Signal Specification1 : SignalSpecification  Unit=km/hr
  Unit Conversion : UnitConversion
  V[mps] : Outport
  wires:
  V[kph]/1 -> Signal Specification1/1
  Unit Conversion/1 -> Signal Specification/1
  Signal Specification1/1 -> Unit Conversion/1
  Signal Specification/1 -> V[mps]/1

== system VehicleDynamics3D_old/Inputs/User Input/Burnout ==
  note: Dummy Variables for Dashboard Instruments
  Burnout : Subsystem  Tag=STV Subsys  LoadFcn=sigbuilder_block('load');  StartFcn=sigbuilder_block('start');  StopFcn=sigbuilder_block('stop');  ClipboardFcn=sigbuilder_block('clipboard');  mask(Sigbuilder block){tuvar=[0:10]}
      mask help: Simulink:masks:SigbuilderBlock_MD
      mask init:
      | if ~strcmp(get_param(bdroot(gcbh),'SimulationStatus'),'stopped') tuvar = sigbuilder_block('maskInit'); end
      settings: CopyFcn=sigbuilder_block('copy');  DeleteFcn=sigbuilder_block('delete');  ModelCloseFcn=sigbuilder_block('modelClose');  PreSaveFcn=sigbuilder_block('preSave');  PauseFcn=sigbuilder_block('pause');  ContinueFcn=sigbuilder_block('continue');  NameChangeFcn=sigbuilder_block('namechange');  OpenFcn=sigbuilder_block('open',[596.4 194.4 550.2 391.8 ]);  CloseFcn=sigbuilder_block('close');
      mask Display: plot(0, 0, 100, 100,[2, 2, 32, 32, 2], [68, 8, 8, 68, 68],[32, 2], [38, 38], [32, 19, 2],[53, 60, 44], [32, 17, 17, 2],[16, 16, 31, 31]);txt = getActiveGroup(gcbh);text(2, 100, txt,'verticalAlignment', 'top');
  Constant1 : Constant  Value=steeringInput
  Constant2 : Constant  Value=vehicleSpeed_kph
  Terminator : Terminator
  Terminator1 : Terminator
  Steering : Outport
  Speed : Outport  Port=2
  wires:
  Burnout/2(Speed) -> Speed/1
  Burnout/1(Steering) -> Steering/1
  Constant1/1 -> Terminator/1
  Constant2/1 -> Terminator1/1

== system VehicleDynamics3D_old/Inputs/User Input/DashboardInput  ==
  Constant1 : Constant  Value=steeringInput
  Constant2 : Constant  Value=vehicleSpeed_kph
  Simulation Pace : aerolibanimutils/Simulation Pace  SimulationPace=1  SleepMode=MATLAB Thread  OutputPaceError=off  SampleTime=SetPaceSampleTime
  Steering : Outport
  Speed : Outport  Port=2
  wires:
  Constant1/1 -> Steering/1
  Constant2/1 -> Speed/1

== system VehicleDynamics3D_old/Inputs/User Input/LeftTurn90 ==
  note: Dummy Variables for Dashboard Instruments
  Constant1 : Constant  Value=steeringInput
  Constant2 : Constant  Value=vehicleSpeed_kph
  LeftTurn : Subsystem  Tag=STV Subsys  LoadFcn=sigbuilder_block('load');  StartFcn=sigbuilder_block('start');  StopFcn=sigbuilder_block('stop');  ClipboardFcn=sigbuilder_block('clipboard');  mask(Sigbuilder block){tuvar=[0:10]}
      mask help: Simulink:masks:SigbuilderBlock_MD
      mask init:
      | if ~strcmp(get_param(bdroot(gcbh),'SimulationStatus'),'stopped') tuvar = sigbuilder_block('maskInit'); end
      settings: CopyFcn=sigbuilder_block('copy');  DeleteFcn=sigbuilder_block('delete');  ModelCloseFcn=sigbuilder_block('modelClose');  PreSaveFcn=sigbuilder_block('preSave');  PauseFcn=sigbuilder_block('pause');  ContinueFcn=sigbuilder_block('continue');  NameChangeFcn=sigbuilder_block('namechange');  OpenFcn=sigbuilder_block('open',[5.4 102.6 1141.2 483.6 ]);  CloseFcn=sigbuilder_block('close');
      mask Display: plot(0, 0, 100, 100,[2, 2, 32, 32, 2], [68, 8, 8, 68, 68],[32, 2], [38, 38], [32, 19, 2],[53, 60, 44], [32, 17, 17, 2],[16, 16, 31, 31]);txt = getActiveGroup(gcbh);text(2, 100, txt,'verticalAlignment', 'top');
  Terminator : Terminator
  Terminator1 : Terminator
  Steering : Outport
  Speed : Outport  Port=2
  wires:
  Constant2/1 -> Terminator1/1
  Constant1/1 -> Terminator/1
  LeftTurn/2(Speed) -> Speed/1
  LeftTurn/1(Steering) -> Steering/1

== system VehicleDynamics3D_old/Inputs/User Input/RightTurn90 ==
  note: Dummy Variables for Dashboard Instruments
  Constant1 : Constant  Value=steeringInput
  Constant2 : Constant  Value=vehicleSpeed_kph
  RightTurn : Subsystem  Tag=STV Subsys  LoadFcn=sigbuilder_block('load');  StartFcn=sigbuilder_block('start');  StopFcn=sigbuilder_block('stop');  ClipboardFcn=sigbuilder_block('clipboard');  mask(Sigbuilder block){tuvar=[0:10]}
      mask help: Simulink:masks:SigbuilderBlock_MD
      mask init:
      | if ~strcmp(get_param(bdroot(gcbh),'SimulationStatus'),'stopped') tuvar = sigbuilder_block('maskInit'); end
      settings: CopyFcn=sigbuilder_block('copy');  DeleteFcn=sigbuilder_block('delete');  ModelCloseFcn=sigbuilder_block('modelClose');  PreSaveFcn=sigbuilder_block('preSave');  PauseFcn=sigbuilder_block('pause');  ContinueFcn=sigbuilder_block('continue');  NameChangeFcn=sigbuilder_block('namechange');  OpenFcn=sigbuilder_block('open',[596.4 225 550.2 361.2 ]);  CloseFcn=sigbuilder_block('close');
      mask Display: plot(0, 0, 100, 100,[2, 2, 32, 32, 2], [68, 8, 8, 68, 68],[32, 2], [38, 38], [32, 19, 2],[53, 60, 44], [32, 17, 17, 2],[16, 16, 31, 31]);txt = getActiveGroup(gcbh);text(2, 100, txt,'verticalAlignment', 'top');
  Terminator : Terminator
  Terminator1 : Terminator
  Steering : Outport
  Speed : Outport  Port=2
  wires:
  Constant1/1 -> Terminator/1
  Constant2/1 -> Terminator1/1
  RightTurn/1(Steering) -> Steering/1
  RightTurn/2(Speed) -> Speed/1

== system VehicleDynamics3D_old/Inputs/User Input/Skidpad ==
  note: Dummy Variables for Dashboard Instruments
  Constant : Constant  Value=24.5
  Constant1 : Constant  Value=steeringInput
  Constant2 : Constant  Value=vehicleSpeed_kph
  Scaling : Gain  Gain=35
  Sine Wave : Sin  Amplitude=15*(pi/180)  Frequency=2*pi*0.05  SampleTime=0
  Terminator : Terminator
  Terminator1 : Terminator
  Steering : Outport
  Speed : Outport  Port=2
  wires:
  Constant/1 -> Speed/1
  Constant2/1 -> Terminator1/1
  Constant1/1 -> Terminator/1
  Scaling/1 -> Steering/1
  Sine Wave/1 -> Scaling/1

== system VehicleDynamics3D_old/Inputs/User Input/Slalom ==
  note: Dummy Variables for Dashboard Instruments
  Constant : Constant  Value=30
  Constant1 : Constant  Value=steeringInput
  Constant2 : Constant  Value=vehicleSpeed_kph
  Scaling : Gain  Gain=10
  Sine Wave : Sin  Amplitude=15*(pi/180)  Frequency=4*pi/10  Phase=pi/2+0.03  SampleTime=0
  Terminator : Terminator
  Terminator1 : Terminator
  Steering : Outport
  Speed : Outport  Port=2
  wires:
  Constant2/1 -> Terminator1/1
  Constant1/1 -> Terminator/1
  Sine Wave/1 -> Scaling/1
  Constant/1 -> Speed/1
  Scaling/1 -> Steering/1

== system VehicleDynamics3D_old/Inputs/User Input/SteepSteer ==
  note: Dummy Variables for Dashboard Instruments
  Constant1 : Constant  Value=steeringInput
  Constant2 : Constant  Value=vehicleSpeed_kph
  SteepSteer : Subsystem  Tag=STV Subsys  LoadFcn=sigbuilder_block('load');  StartFcn=sigbuilder_block('start');  StopFcn=sigbuilder_block('stop');  ClipboardFcn=sigbuilder_block('clipboard');  mask(Sigbuilder block){tuvar=[0:10]}
      mask help: Simulink:masks:SigbuilderBlock_MD
      mask init:
      | if ~strcmp(get_param(bdroot(gcbh),'SimulationStatus'),'stopped') tuvar = sigbuilder_block('maskInit'); end
      settings: CopyFcn=sigbuilder_block('copy');  DeleteFcn=sigbuilder_block('delete');  ModelCloseFcn=sigbuilder_block('modelClose');  PreSaveFcn=sigbuilder_block('preSave');  PauseFcn=sigbuilder_block('pause');  ContinueFcn=sigbuilder_block('continue');  NameChangeFcn=sigbuilder_block('namechange');  OpenFcn=sigbuilder_block('open',[342.6 225 550.8 361.2 ]);  CloseFcn=sigbuilder_block('close');
      mask Display: plot(0, 0, 100, 100,[2, 2, 32, 32, 2], [68, 8, 8, 68, 68],[32, 2], [38, 38], [32, 19, 2],[53, 60, 44], [32, 17, 17, 2],[16, 16, 31, 31]);txt = getActiveGroup(gcbh);text(2, 100, txt,'verticalAlignment', 'top');
  Terminator : Terminator
  Terminator1 : Terminator
  Steering : Outport
  Speed : Outport  Port=2
  wires:
  Constant1/1 -> Terminator/1
  Constant2/1 -> Terminator1/1
  SteepSteer/2(Speed) -> Speed/1
  SteepSteer/1(Steering) -> Steering/1
